simulink model "Phase1"  (R2022b)
settings: Solver=ode4  StartTime=0  StopTime=15  FixedStep=0.001  RelTol=1e-3
InitFcn:
  | initialize;
StopFcn:
  | ending;
values from neighbouring files (symbols this model uses):
  g = 9.81    [initialize.m]
undefined symbols (not defined in the file or in its folder): body, chi0, lambda0, omega0, RRV, v0
libraries: shared6dof x1, sharedtransform x1, uavutilslib x1
settings Model: Creator=farha  LastModifiedBy=Alire
settings SolverCC: AlgebraicLoopSolver=TrustRegion
settings DebuggingCC: UnconnectedInputMsg=warning  UnconnectedOutputMsg=warning  UnconnectedLineMsg=warning  SFMachineParentedDataDiag=warning
settings ModelReferenceCC: EnableRefExpFcnMdlSchedulingChecks=on
settings RTWCC: DLArmComputeVersion=19.05

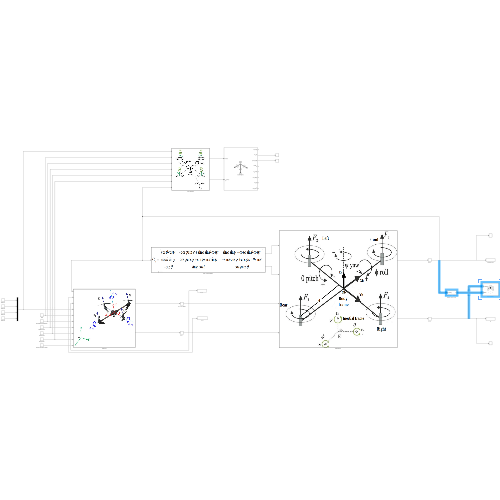
[thumbnail: Simulink's stored preview of the top-level diagram]
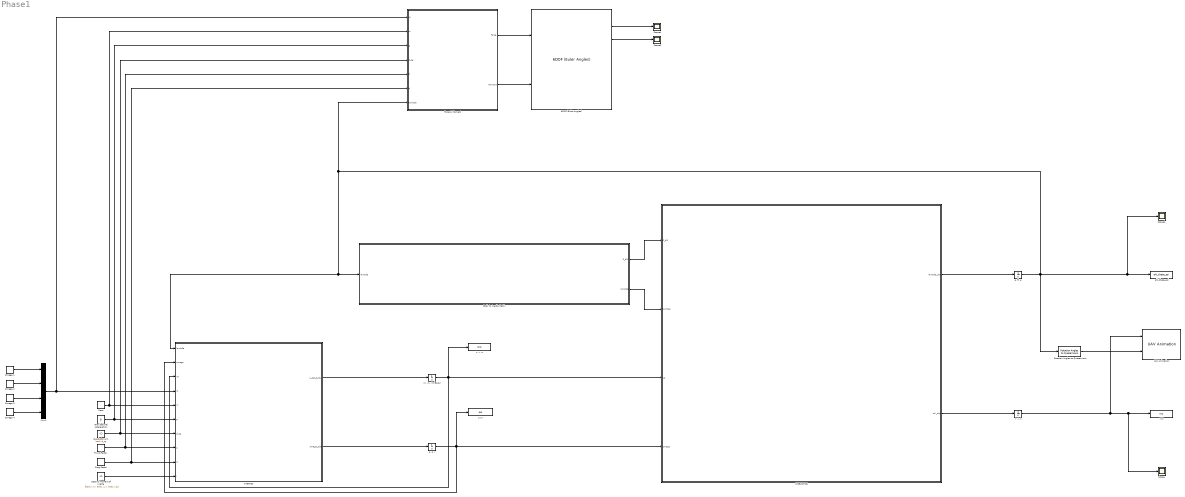
== system Phase1 ==
  6DOF (Euler Angles) : shared6dof/6DOF (Euler Angles)  units=Metric (MKS)  mtype=Fixed  rep=Euler Angles  xme_0=[chi0.x; chi0.y; chi0.z]  Vm_0=[v0.x; v0.y; v0.z]  eul_0=[lambda0.phi; lambda0.theta; lambda0.psi]  pm_0=[omega0.p; omega0.q; omega0.r]  mass_0=body.m  mass_e=0.5  mass_f=2.0  inertia=[body.I.xx 0 0; 0 body.I.yy 0; 0 0 body.I.zz]  inertia_e=eye(3)  inertia_f=2*eye(3)  k_quat=1.0  vre_flag=on  abi_flag=off  aMode=0  xme_statename=''  Vm_statename=''  eul_statename=''  quat_statename=''  pm_statename=''  mass_statename=''
  Body to Inertia Matrix : MATLAB Function  TreatAsAtomicUnit=on
  Drag Factor : Constant  Value=body.d
  Force & Moment : MATLAB Function  TreatAsAtomicUnit=on
  Gravitational Acceleration : Constant  Value=g
  KINEMATICS : MATLAB Function  TreatAsAtomicUnit=on
  KINETICS : MATLAB Function  TreatAsAtomicUnit=on
  Mass : Constant  Value=body.m
  Mux1 : Mux
  Omega 1 : Constant  Value=RRV.R1
  Omega 2 : Constant  Value=RRV.R2
  Omega 3 : Constant  Value=RRV.R3
  Omega 4 : Constant  Value=RRV.R4
  Quadrotor Arm : Constant  Value=body.d_cg
  Rotation Angles to Quaternions : sharedtransform/Rotation Angles to Quaternions  rotationOrder=ZYX  aMode=aMode
  Scope{,1..2,4} (4 alike) : Scope
  Second moment of inertia : Constant  Value=[body.I.xx; body.I.yy; body.I.zz]
  Thrust Factor : Constant  Value=body.b
  UAV Animation : uavutilslib/UAV Animation  UAVType=Multirotor  UAVSize=1  InertialZDirection=Down  SampleTime=-1
  "Vx, Vy, Vz (Body)" : Integrator  InitialCondition=[v0.x; v0.y; v0.z]
  p q r : ToWorkspace  VariableName=pqr  SampleTime=-1
  "p, q, r" : Integrator  InitialCondition=[omega0.p; omega0.q; omega0.r]
  phi_theta_psi : ToWorkspace  VariableName=phi_theta_psi  SampleTime=-1
  "u, v, w" : ToWorkspace  VariableName=uvw  SampleTime=-1
  "x, y, z" : Integrator  InitialCondition=[chi0.x; chi0.y; chi0.z]
  xyz : ToWorkspace  VariableName=xyz  SampleTime=-1
  "φ, θ, ψ" : Integrator  InitialCondition=[lambda0.phi; lambda0.theta; lambda0.psi]
  wires:
  Body to Inertia Matrix/1(C_b2i) -> KINEMATICS/1(C_b2i)
  Body to Inertia Matrix/2(lambda) -> KINEMATICS/2(lambda)
  Omega 2/1 -> Mux1/2
  Omega 1/1 -> Mux1/1
  Omega 4/1 -> Mux1/4
  Omega 3/1 -> Mux1/3
  Mux1/1 -> KINETICS/4(W), Force & Moment/1(W)
  KINETICS/2(omega_dot) -> "p, q, r"/1
  "p, q, r"/1 -> p q r/1, KINETICS/2(omega), KINEMATICS/4(omega)
  Second moment of inertia/1 -> KINETICS/10(I)
  Gravitational Acceleration/1 -> KINETICS/6(g), Force & Moment/3(g)
  Mass/1 -> KINETICS/5(m), Force & Moment/2(m)
  Quadrotor Arm/1 -> Force & Moment/4(d_cg), KINETICS/7(d_cg)
  Thrust Factor/1 -> KINETICS/8(b), Force & Moment/5(b)
  Drag Factor/1 -> KINETICS/9(d), Force & Moment/6(d)
  KINEMATICS/2(chi_dot) -> "x, y, z"/1
  KINEMATICS/1(lambda_dot) -> "φ, θ, ψ"/1
  KINETICS/1(V_dot_body) -> "Vx, Vy, Vz (Body)"/1
  "Vx, Vy, Vz (Body)"/1 -> "u, v, w"/1, KINEMATICS/3(Vb), KINETICS/3(Vb)
  "x, y, z"/1 -> Scope/1, xyz/1, UAV Animation/1
  "φ, θ, ψ"/1 -> Rotation Angles to Quaternions/1, Scope1/1, phi_theta_psi/1, Force & Moment/7(lambda), KINETICS/1(lambda), Body to Inertia Matrix/1("lambda ")
  Rotation Angles to Quaternions/1 -> UAV Animation/2
  Force & Moment/1(Force) -> 6DOF (Euler Angles)/1
  Force & Moment/2(Moment) -> 6DOF (Euler Angles)/2
  6DOF (Euler Angles)/3 -> Scope2/1
  6DOF (Euler Angles)/2 -> Scope4/1

== matlab function Phase1/Body to Inertia Matrix ==
  data: lambda input; C_b2i output; lambda output
function [C_b2i, lambda] = fcn(lambda)
phi = lambda(1);
theta = lambda(2);
psi = lambda(3);
C_b2i = [cos(theta)*cos(psi), -cos(phi)*sin(psi)+sin(phi)*sin(theta)*cos(psi), sin(phi)*sin(psi)+cos(phi)*sin(theta)*cos(psi);
         cos(theta)*sin(psi),  cos(phi)*cos(psi)+sin(phi)*sin(theta)*sin(psi),-sin(phi)*cos(psi)+cos(phi)*sin(theta)*sin(psi);
        -sin(theta)         ,  sin(phi)*cos(theta)                           , cos(phi)*cos(theta)                          ];

== matlab function Phase1/KINEMATICS ==
  data: lambda_dot output; C_b2i input; lambda input; chi_dot output; Vb input; omega input
function [lambda_dot, chi_dot] = fcn(C_b2i, lambda, Vb, omega)
chi_dot = C_b2i*Vb;
omega2lamda_dot = [1, sin(lambda(1))*tan(lambda(2)), cos(lambda(1))*tan(lambda(2));
                   0, cos(lambda(1))               , -sin(lambda(1))              ;
                   0, sin(lambda(1))/cos(lambda(2)), cos(lambda(1))/cos(lambda(2))];
lambda_dot = omega2lamda_dot*omega;

== matlab function Phase1/KINETICS ==
  data: lambda input; omega input; Vb input; W input; m input; g input; d_cg input; b input; d input; V_dot_body output; I input; omega_dot output
function [V_dot_body, omega_dot] = fcn(lambda, omega, Vb, W, m, g, d_cg, b, d, I)
% initializing
Ixx = I(1); Iyy = I(2); Izz = I(3);
phi = lambda(1); theta = lambda(2);
p = omega(1); q = omega(2); r = omega(3);
u = Vb(1); v = Vb(2); w = Vb(3);
% Creating V_dot_body
udot = r*v - q*w - g*sin(theta);
vdot = p*w - r*u + g*cos(theta)*sin(phi);
wdot =  - (b*W(1)^2 + b*W(2)^2 + b*W(3)^2 + b*W(4)^2 + m*(p*v - q*u) - g*m*cos(phi)*cos(theta))/m;
V_dot_body = [udot; vdot; wdot];

% Creating omega_dot
pdot = (b*d_cg*(W(2)^2 - W(4)^2) + q*r*(Iyy - Izz))/Ixx;
qdot = (b*d_cg*(W(1)^2 - W(3)^2) - p*r*(Ixx - Izz))/Iyy;
rdot = (d*(W(1)^2 - W(2)^2 + W(3)^2 - W(4)^2) + p*q*(Ixx - Iyy))/Izz;
omega_dot = [pdot; qdot; rdot];

== matlab function Phase1/Force & Moment ==
  data: W input; m input; g input; d_cg input; b input; d input; lambda input; Force output; Moment output
function [Force, Moment] = fcn(W, m, g, d_cg, b, d, lambda)
% Forces
Fx = -m*g*sin(lambda(2));
Fy = m*g*sin(lambda(1))*cos(lambda(2));
Fz = m*g*cos(lambda(1))*cos(lambda(2)) - b*(W(1)^2 + W(2)^2 + W(3)^2 + W(4)^2);
Force = [Fx; Fy; Fz];
% Moments
Mx = d_cg*b*(W(2)^2 - W(4)^2);
My = d_cg*b*(W(1)^2 - W(3)^2);
Mz = d*(W(1)^2 + W(3)^2 - W(2)^2 - W(4)^2);
Moment = [Mx; My; Mz];
